simulink model "Mdl_11_CloseLoop_Discrete"  (R2018a)
settings: Solver=VariableStepAuto  StartTime=0.0  StopTime=10.0  RelTol=1e-3
undefined symbols (not defined in the file): A_mdl, B_mdl, C_mdl, D_mdl, K_mdl, simSwitch, Ts
settings Model: Creator=pala  LastModifiedBy=pala
settings DataIOCC: SaveFinalState=on  SaveFormat=StructureWithTime  SaveState=on  SignalLogging=off  DSMLogging=off

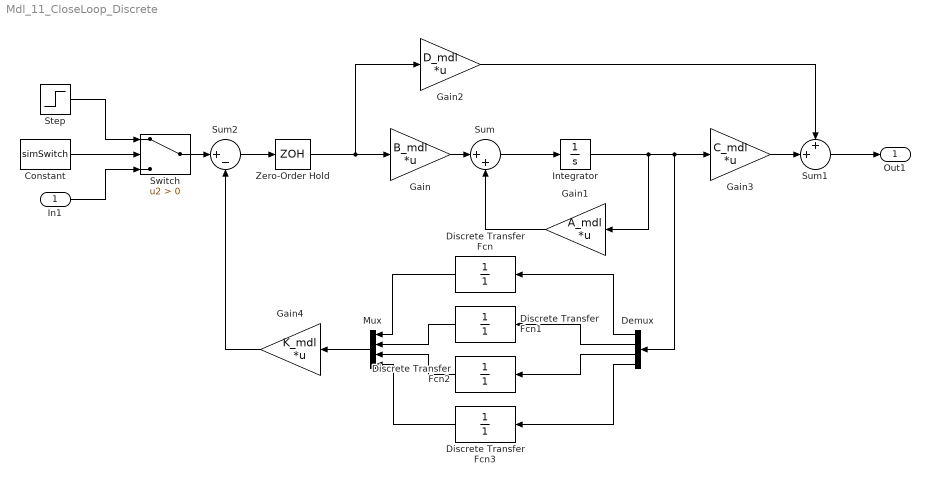
== system Mdl_11_CloseLoop_Discrete ==
  In1 : Inport
  Constant : Constant  Value=simSwitch
  Demux : Demux
  Discrete Transfer Fcn{,1..3} (4 alike) : DiscreteTransferFcn  Denominator=[1]  SampleTime=Ts
  Gain : Gain  Gain=B_mdl  Multiplication=Matrix(K*u)
  Gain1 : Gain  Gain=A_mdl  Multiplication=Matrix(K*u)
  Gain2 : Gain  Gain=D_mdl  Multiplication=Matrix(K*u)
  Gain3 : Gain  Gain=C_mdl  Multiplication=Matrix(K*u)
  Gain4 : Gain  Gain=K_mdl  Multiplication=Matrix(K*u)
  Integrator : Integrator
  Mux : Mux
  Step : Step  SampleTime=0
  Sum : Sum  Inputs=|++
  Sum1 : Sum  Inputs=++|
  Sum2 : Sum  Inputs=|+-
  Switch : Switch  Criteria=u2 > Threshold
  Zero-Order Hold : ZeroOrderHold  SampleTime=Ts
  Out1 : Outport
  wires:
  Step/1 -> Switch/1
  In1/1 -> Switch/3
  Constant/1 -> Switch/2
  Gain/1 -> Sum/1
  Gain1/1 -> Sum/2
  Sum/1 -> Integrator/1
  Integrator/1 -> Gain1/1, Demux/1, Gain3/1
  Gain2/1 -> Sum1/1
  Gain3/1 -> Sum1/2
  Sum1/1 -> Out1/1
  Gain4/1 -> Sum2/2
  Switch/1 -> Sum2/1
  Sum2/1 -> Zero-Order Hold/1
  Demux/1 -> Discrete Transfer Fcn/1
  Demux/2 -> Discrete Transfer Fcn1/1
  Demux/3 -> Discrete Transfer Fcn2/1
  Demux/4 -> Discrete Transfer Fcn3/1
  Mux/1 -> Gain4/1
  Discrete Transfer Fcn/1 -> Mux/1
  Discrete Transfer Fcn1/1 -> Mux/2
  Discrete Transfer Fcn2/1 -> Mux/3
  Discrete Transfer Fcn3/1 -> Mux/4
  Zero-Order Hold/1 -> Gain2/1, Gain/1
